simulink model "motion_cue"  (R2014b)
settings: Solver=VariableStepAuto  StartTime=0.0  StopTime=5  FixedStep=.001  MaxStep=.01  RelTol=1e-3
libraries: simulink x1
settings Model: Creator=brownlab  LastModifiedBy=brownaa
settings DataIOCC: SaveFormat=Dataset
settings OptimizationCC: UseDivisionForNetSlopeComputation=off  SimCompilerOptimization=off
settings DebuggingCC: SolverPrmCheckMsg=none  FrameProcessingCompatibilityMsg=error  AllowSymbolicDim=off
settings HardwareCC: ProdBitPerPointer=64  ProdLargestAtomicFloat=Float  ProdIntDivRoundTo=Zero  ProdEndianess=LittleEndian  ProdWordSize=64  ProdHWDeviceType=Intel->x86-64 (Windows64)
settings RTWCC: RTWCompilerOptimization=off
settings GRTTargetCC: GeneratePreprocessorConditionals=Use local settings
settings ConfigComp: CovMetricSettings=dw  CovHtmlReporting=on  CovSaveCumulativeToWorkspaceVar=on  CovSaveSingleToWorkspaceVar=on  CovExternalEMLEnable=off

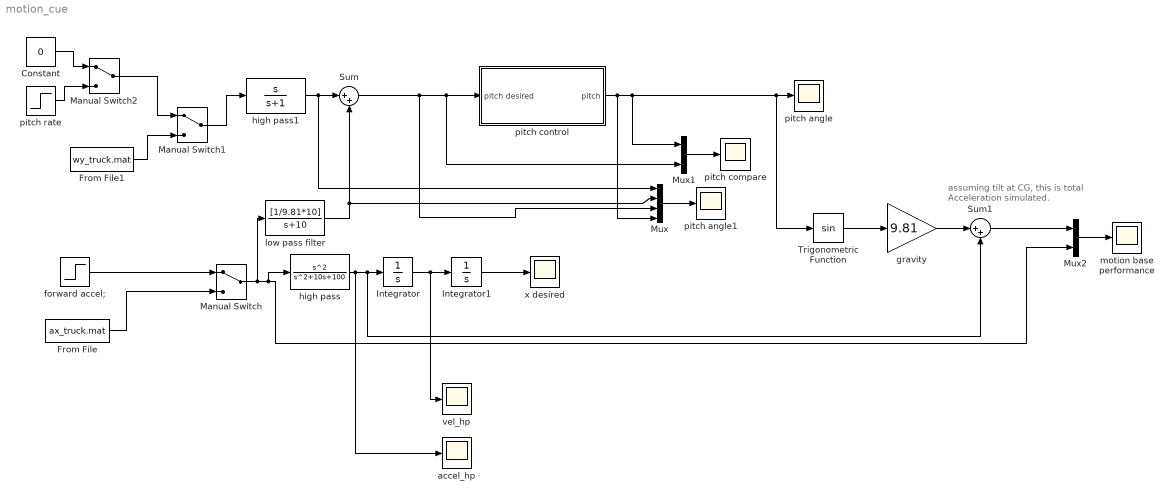
== system motion_cue ==
  note: assuming tilt at CG, this is total
      | Acceleration simulated.
  Constant : Constant  Value=0
  From File : FromFile  FileName=ax_truck.mat  SampleTime=0
  From File1 : FromFile  FileName=wy_truck.mat  SampleTime=0
  Integrator : Integrator
  Integrator1 : Integrator
  Manual Switch : ManualSwitch
  Manual Switch1 : ManualSwitch
  Manual Switch2 : ManualSwitch
  Mux : Mux
  Mux1 : Mux  Inputs=2
  Mux2 : Mux  Inputs=2
  Sum : Sum  Inputs=|++
  Sum1 : Sum  Inputs=|++
  Trigonometric Function : Trigonometry
  accel_hp : Scope
      settings: YMin=-0.04644  YMax=1.06739  SaveName=ScopeData7
  forward accel; : Step  SampleTime=0
  gravity : Gain  Gain=9.81
  high pass : TransferFcn  Numerator=[1 0 0]  Denominator=[1 10 100]
  high pass1 : TransferFcn  Numerator=[1 0]  Denominator=[1 1]
  low pass filter : TransferFcn  Numerator=[1/9.81*10]  Denominator=[1 10]
  motion base performance : Scope
      settings: YMin=-0.04644  YMax=1.06739  SaveName=ScopeData5
  pitch angle : Scope
      settings: YMin=-0.04644  YMax=1.06739
  pitch angle1 : Scope
      settings: YMin=-0.1508  YMax=0.11129
  pitch compare : Scope
      settings: YMin=-0.1449  YMax=0.0582  SaveName=ScopeData4
  pitch control : Subsystem
  pitch rate : Step  SampleTime=0
  "vel_hp " : Scope
      settings: YMin=-0.04644  YMax=1.06739  SaveName=ScopeData6
  x desired : Scope
      settings: YMin=-0.04644  YMax=1.06739  SaveName=ScopeData2
  wires:
  pitch control/1(pitch) -> Mux/4, Mux1/1, Trigonometric Function/1, pitch angle/1
  Integrator/1 -> "vel_hp "/1, Integrator1/1
  Integrator1/1 -> x desired/1
  low pass filter/1 -> Mux/2, Sum/2
  high pass1/1 -> Mux/1, Sum/1
  Sum/1 -> Mux/3, Mux1/2, pitch control/1("pitch desired ")
  Mux/1 -> pitch angle1/1
  forward accel;/1 -> Manual Switch/1
  From File/1 -> Manual Switch/2
  From File1/1 -> Manual Switch1/2
  Manual Switch1/1 -> high pass1/1
  Mux1/1 -> pitch compare/1
  Constant/1 -> Manual Switch2/1
  pitch rate/1 -> Manual Switch2/2
  Manual Switch2/1 -> Manual Switch1/1
  Trigonometric Function/1 -> gravity/1
  gravity/1 -> Sum1/1
  high pass/1 -> accel_hp/1, Sum1/2, Integrator/1
  Sum1/1 -> Mux2/1
  Manual Switch/1 -> low pass filter/1, Mux2/2, high pass/1
  Mux2/1 -> motion base performance/1

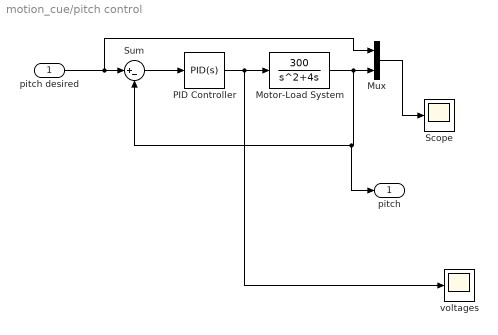
== system motion_cue/pitch control ==
  "pitch desired " : Inport
  Motor-Load System : TransferFcn  Numerator=[300]  Denominator=[1 4 0]
  Mux : Mux  Inputs=2
  PID Controller : simulink/Continuous/PID Controller  Controller=PID  TimeDomain=Continuous-time  SampleTime=-1  IntegratorMethod=Forward Euler  FilterMethod=Forward Euler  Form=Parallel  P=1  I=0  D=.1  N=100  InitialConditionSource=internal  InitialConditionForIntegrator=0  InitialConditionForFilter=0  ExternalReset=none  LimitOutput=off  UpperSaturationLimit=inf  LowerSaturationLimit=-inf  LinearizeAsGain=on  AntiWindupMode=none  Kb=1  TrackingMode=off  Kt=1  PParamMin=[]  PParamMax=[]  IParamMin=[]  IParamMax=[]  DParamMin=[]  DParamMax=[]  NParamMin=[]  NParamMax=[]  KbParamMin=[]  KbParamMax=[]  KtParamMin=[]  KtParamMax=[]  POutMin=[]  POutMax=[]  IOutMin=[]  IOutMax=[]  DOutMin=[]  DOutMax=[]  NOutMin=[]  NOutMax=[]  KbOutMin=[]  KbOutMax=[]  KtOutMin=[]  KtOutMax=[]  IntegratorOutMin=[]  IntegratorOutMax=[]  FilterOutMin=[]  FilterOutMax=[]  SumOutMin=[]  SumOutMax=[]  SumI1OutMin=[]  SumI1OutMax=[]  SumI2OutMin=[]  SumI2OutMax=[]  SumI3OutMin=[]  SumI3OutMax=[]  SumDOutMin=[]  SumDOutMax=[]  SaturationOutMin=[]  SaturationOutMax=[]  IntegratorContinuousStateAttributes=''  IntegratorStateMustResolveToSignalObject=off  IntegratorRTWStateStorageClass=Auto  FilterContinuousStateAttributes=''  FilterStateMustResolveToSignalObject=off  FilterRTWStateStorageClass=Auto  DifferentiatorICPrevScaledInput=0  DifferentiatorOutMin=[]  DifferentiatorOutMax=[]  UseFilter=on
  Scope : Scope
  Sum : Sum  Inputs=|+-
  voltages : Scope
      settings: YMin=-0.07925  YMax=1.03576  SaveName=ScopeData3
  pitch : Outport
  wires:
  PID Controller/1 -> voltages/1, Motor-Load System/1
  "pitch desired "/1 -> Mux/1, Sum/1
  Sum/1 -> PID Controller/1
  Motor-Load System/1 -> pitch/1, Sum/2, Mux/2
  Mux/1 -> Scope/1
